simulink model "SD2231_Lab1_2022"  (R2020b)
settings: Solver=VariableStepAuto  StartTime=0.0  StopTime=inf  RelTol=1e-3
values from neighbouring files (symbols this model uses):
  delay = 250    [initial.m]
  K_awup = Ki_br_r/Kp_br_r    (= 10.4166666667)    [initial.m]
  K_brake = K_brake(3)    [initial.m]
  K_em = K_em(3)    [initial.m]
  Kd_br_f = 0*0.6*T_new_rl_b    (= 0)    [initial.m]
  Kd_br_r = 0.6*T_new_rl_b    (= 0.1722)    [initial.m]
  Kd_tr = 0.6*T_new    (= 0.0093)    [initial.m]
  Ki_br_f = 0.5*0.6*T_new_rl_b/L_new_rl_b^2    (= 37.3697916667)    [initial.m]
  Ki_br_r = 0.6*T_new_rl_b/L_new_rl_b^2    (= 74.7395833333)    [initial.m]
  Ki_tr = 0.6*T_new/L_new^2    (= 4.12188365651)    [initial.m]
  Kp_br_f = 1.2*T_new_rl_b/L_new_rl_b    (= 7.175)    [initial.m]
  Kp_br_r = 1.2*T_new_rl_b/L_new_rl_b    (= 7.175)    [initial.m]
  Kp_tr = 2.2*1.2*T_new/L_new    (= 0.861473684211)    [initial.m]
  N = 100    [initial.m]
  ref_br_f = 0.15    [initial.m]
  ref_br_r = 0.17-0.1    (= 0.07)    [initial.m]
  ref_tr = 0.06    [initial.m]
  step_time = 2    [initial.m]
  threshold_br_f = ref_br_f-0.05    (= 0.1)    [initial.m]
  threshold_br_r = ref_br_r-0.05    (= 0.02)    [initial.m]
  threshold_tc = ref_tr-0.02    (= 0.04)    [initial.m]
  vx_threshold = 1    [initial.m]
undefined symbols (not defined in the file or in its folder): DiscIntNeverNeededParam, Veh
libraries: CarMaker4SL x38, simulink x2, autolibmappedmotor x2
(part 1 of 4)
settings Model: Creator=Edwin solomon  LastModifiedBy=rivaa

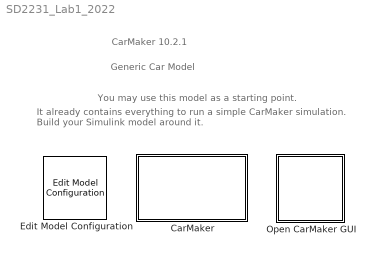
== system SD2231_Lab1_2022 ==
  note: You may use this model as a starting point.
  note: CarMaker 10.2.1
  note: It already contains everything to run a simple CarMaker simulation.
      | Build your Simulink model around it.
  note: Generic Car Model
  CarMaker : Subsystem  TreatAsAtomicUnit=on
      mask Display: image(imread('CarMakerSys.png'));
  Edit Model Configuration : CarMaker4SL/Edit Model Configuration  SFunctionModules=''
  Open CarMaker GUI : Subsystem  LoadFcn=if ~length(which('cmself')), cmenv; end
      settings: OpenFcn=cmblockmagic('gui_fix_display'); CM_Simulink
      mask Display: image(imread('CarMakerGUI.png'));

== system SD2231_Lab1_2022/CarMaker ==
  Bus Creator : BusCreator  Inputs=6
  CM_FIRST : Subsystem
  CM_LAST : Subsystem
  CarMaker data : Subsystem
  DrivMan : Subsystem
  Ground : Ground
  IPG Vehicle : Subsystem  TreatAsAtomicUnit=on
  Road friction : Subsystem
      settings: PortSchema="{\"entries\":[{\"content\":{\"sides\":[{\"content\":{\"connectorIds\":[]},\"type\":\"ConnectorPlacement.EquallySpacedRectSide\",\"uuid\":\"1e02911d-bb16-4af8-b063-0b1c76ab284f\"},{\"content\":{\"connectorIds\":[],\"side\":\"RIGHT\"},\"type\":\"ConnectorPlacement.EquallySpacedRectSide\",\"uuid\":\"1455e6df-1fb8-405b-9b14-078dc452472c\"},{\"content\":{\"connectorIds\":[\"In1\"],\"side\":\"TOP\"},\"type\":\"ConnectorPlacement.EquallySpacedRectSide\",\"uuid\":\"c8dda622-f685-4f5f-94e7-d49e41573b19\"},{\"content\":{\"connectorIds\":[],\"side\":\"HIDDEN\"},\"type\":\"ConnectorPlacement.EquallySpacedRectSide\",\"uuid\":\"9a4d84ea-b740-4dd8-ac4f-aa27e6a4f3a4\"}]},\"type\":\"ConnectorPlacement.EquallySpacedConnector\",\"uuid\":\"f3a55054-1857-4c4c-b5da-0ded36d4ade6\"}],\"packageUris\":[\"http://schema.mathworks.com/mf0/Connector/R2020b\"],\"version\":\"1.0\"}"
  Terminator : Terminator
  Used friction mapping : Subsystem
  VehicleControl : Subsystem
  Your ABS Controller : Subsystem
  Your Traction Controller : Subsystem
  Your observer : Subsystem
  wires:
  DrivMan/2(DrivMan.Out) -> VehicleControl/2(DrivMan.In)
  DrivMan/1(Sync_Out) -> VehicleControl/1(Sync_In)
  CM_FIRST/2(Env.Misc) -> DrivMan/2(Env.Misc)
  CM_FIRST/1(Sync_Out) -> DrivMan/1(Sync_In)
  CM_LAST/1(Sync_Out) -> Terminator/1
  Ground/1 -> CM_FIRST/1(Sync_In)
  IPG Vehicle/1(Sync_Out) -> CM_LAST/1(Sync_In)
  VehicleControl/1(Sync_Out) -> IPG Vehicle/1(Sync_In)
  VehicleControl/3(VhclCtrl.Steering) -> IPG Vehicle/3(VhclCtrl.Steering)
  VehicleControl/4(Vhcl.Wheel.In) -> IPG Vehicle/4(Vhcl.Wheel.In)
  VehicleControl/5(Vhcl.Misc) -> IPG Vehicle/5(Vhcl.Misc)
  VehicleControl/6(VhclCtrl.Brake) -> IPG Vehicle/6(VhclCtrl.Brake)
  VehicleControl/7(VhclCtrl.PT) -> IPG Vehicle/7(VhclCtrl.PT)
  VehicleControl/2(Vhcl.Model.Source) -> IPG Vehicle/2(Vhcl.Model.Source)
  Your Traction Controller/2(RR TrqReqSignal (0-1)) -> Bus Creator/2
  Your observer/2(Tyre slip bus data out) -> Your Traction Controller/2(Tyre slip bus data out), Used friction mapping/1(Tyre slip bus data out), Your ABS Controller/2(Tyre slip bus data out)
  Your observer/1(CarMaker bus data out) -> Your Traction Controller/1(CarMaker Bus data), Your ABS Controller/1(CarMaker Bus data)
  Your ABS Controller/3(RLBrakeAdjust (0-1)) -> Bus Creator/5
  CarMaker data/1(CarMaker bus data) -> Your observer/1(CarMaker bus data), Road friction/1(CarMaker bus data)
  Your ABS Controller/1(FLBrakeAdjust (0-1)) -> Bus Creator/3
  Your Traction Controller/1(LR TrqReqSignal (0-1)) -> Bus Creator/1
  Your ABS Controller/4(RRBrakeAdjust (0-1)) -> Bus Creator/6
  Bus Creator/1 -> IPG Vehicle/8(SD2231.data)
  Your ABS Controller/2(FRBrakeAdjust (0-1)) -> Bus Creator/4

== system SD2231_Lab1_2022/Open CarMaker GUI ==
  S-Function : S-Function  FunctionName=cm_gui  SFunctionDeploymentMode=off  EnableBusSupport=off

== system SD2231_Lab1_2022/CarMaker/CM_FIRST ==
  Sync_In : Inport
  BusCreator1 : BusCreator  Inputs=8
  BusCreator2 : BusCreator  Inputs=6
  Demux1 : Demux  Outputs=14
      settings: DisplayOption=none
  Environment : S-Function  FunctionName=CM_Sfun  Parameters='Environment'  SFunctionDeploymentMode=off  EnableBusSupport=off
  IoIn : S-Function  FunctionName=CM_Sfun  Parameters='IoIn'  SFunctionDeploymentMode=off  EnableBusSupport=off
  Terminator : Terminator
  Sync_Out : Outport
  Env.Misc : Outport  Port=2
  wires:
  BusCreator2/1 -> Terminator/1  "IF Environment (in)"
  BusCreator1/1 -> Env.Misc/1
  Demux1/14 -> BusCreator2/6  "Env sRoad"
  Demux1/13 -> BusCreator2/5  "Env PoI_GCS Elev"
  Demux1/12 -> BusCreator2/4  "Env PoI_GCS Lat"
  Demux1/11 -> BusCreator2/3  "Env PoI_GCS Long"
  Demux1/10 -> BusCreator2/2  "Env Time"
  Demux1/9 -> BusCreator2/1  "Env yDay"
  Demux1/8 -> BusCreator1/8  "Env WindVel_tot z"
  Demux1/7 -> BusCreator1/7  "Env WindVel_tot y"
  Demux1/6 -> BusCreator1/6  "Env WindVel_tot x"
  Demux1/5 -> BusCreator1/5  "Env SolarRadiation"
  Demux1/4 -> BusCreator1/4  "Env AirHumidity"
  Demux1/3 -> BusCreator1/3  "Env AirPressure"
  Demux1/2 -> BusCreator1/2  "Env AirDensity"
  Demux1/1 -> BusCreator1/1  "Env Temperature"
  Environment/2 -> Demux1/1
  Environment/1 -> Sync_Out/1
  IoIn/1 -> Environment/1
  Sync_In/1 -> IoIn/1

== system SD2231_Lab1_2022/CarMaker/CM_LAST ==
  Sync_In : Inport
  CM_User : S-Function  FunctionName=CM_Sfun  Parameters='CM_User'  SFunctionDeploymentMode=off  EnableBusSupport=off
  IoOut : S-Function  FunctionName=CM_Sfun  Parameters='IoOut'  SFunctionDeploymentMode=off  EnableBusSupport=off
  Sync_Out : Outport
  wires:
  IoOut/1 -> Sync_Out/1
  CM_User/1 -> IoOut/1
  Sync_In/1 -> CM_User/1

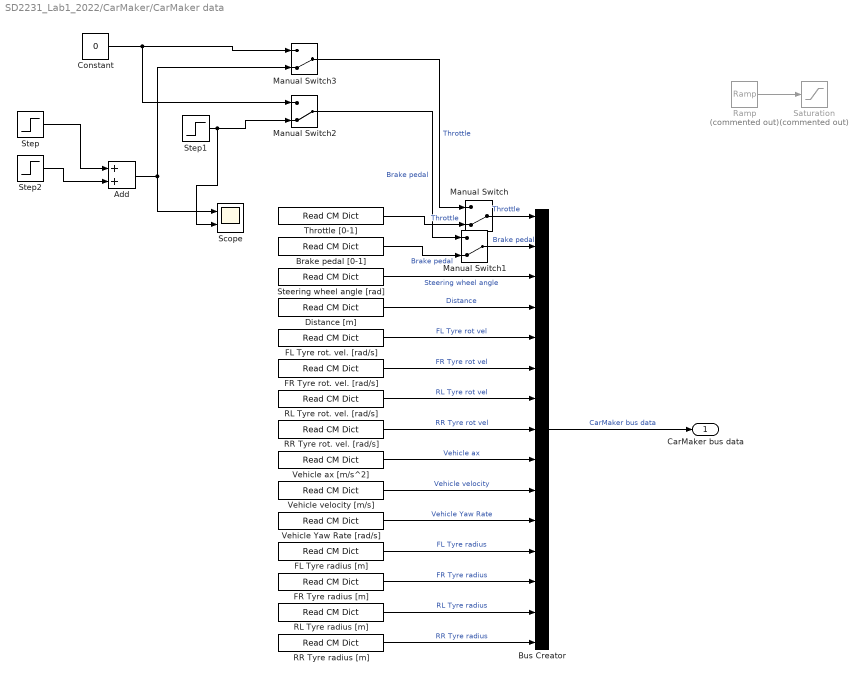
== system SD2231_Lab1_2022/CarMaker/CarMaker data ==
  Add : Sum
  Brake pedal [0-1] : CarMaker4SL/Read CM Dict  xname=Driver.Brake  xsync=off  xstime=Continuous
  Bus Creator : BusCreator  Inputs=15
  Constant : Constant  Value=0
  Distance [m] : CarMaker4SL/Read CM Dict  xname=Vhcl.Distance  xsync=off  xstime=Continuous
  FL Tyre radius [m] : CarMaker4SL/Read CM Dict  xname=Car.WFL.Radius  xsync=off  xstime=Continuous
  FL Tyre rot. vel. [rad/s] : CarMaker4SL/Read CM Dict  xname=Car.WheelSpd_FL  xsync=off  xstime=Continuous
  FR Tyre radius [m] : CarMaker4SL/Read CM Dict  xname=Car.WFR.Radius  xsync=off  xstime=Continuous
  FR Tyre rot. vel. [rad/s] : CarMaker4SL/Read CM Dict  xname=Car.WheelSpd_FR  xsync=off  xstime=Continuous
  Manual Switch{,1..3} (4 alike) : ManualSwitch  CurrentSetting=0
  RL Tyre radius [m] : CarMaker4SL/Read CM Dict  xname=Car.WRL.Radius  xsync=off  xstime=Continuous
  RL Tyre rot. vel. [rad/s] : CarMaker4SL/Read CM Dict  xname=Car.WheelSpd_RL  xsync=off  xstime=Continuous
  RR Tyre radius [m] : CarMaker4SL/Read CM Dict  xname=Car.WRR.Radius  xsync=off  xstime=Continuous
  RR Tyre rot. vel. [rad/s] : CarMaker4SL/Read CM Dict  xname=Car.WheelSpd_RR  xsync=off  xstime=Continuous
  Ramp : simulink/Sources/Ramp  Commented=on  slope=1/0.1  start=step_time  InitialOutput=0
  Saturation : Saturate  Commented=on  UpperLimit=1  LowerLimit=0
  Scope : Scope  NumInputPorts=2
  Steering wheel angle [rad] : CarMaker4SL/Read CM Dict  xname=Driver.Steer.Ang  xsync=off  xstime=Continuous
  Step : Step  Time=step_time  SampleTime=0
  Step1 : Step  Time=step_time + 6  SampleTime=0
  Step2 : Step  Time=step_time + 3  After=-1  SampleTime=0
  Throttle [0-1] : CarMaker4SL/Read CM Dict  xname=Driver.Gas  xsync=off  xstime=Continuous
  Vehicle Yaw Rate [rad/s] : CarMaker4SL/Read CM Dict  xname=Car.YawRate  xsync=off  xstime=Continuous
  Vehicle ax [m/s^2] : CarMaker4SL/Read CM Dict  xname=Car.ax  xsync=off  xstime=Continuous
  Vehicle velocity [m/s] : CarMaker4SL/Read CM Dict  xname=Car.v  xsync=off  xstime=Continuous
  CarMaker bus data : Outport  VectorParamsAs1DForOutWhenUnconnected=off
  wires:
  RR Tyre rot. vel. [rad/s]/1 -> Bus Creator/8  "RR Tyre rot vel"
  RL Tyre rot. vel. [rad/s]/1 -> Bus Creator/7  "RL Tyre rot vel"
  Distance [m]/1 -> Bus Creator/4  "Distance"
  FR Tyre rot. vel. [rad/s]/1 -> Bus Creator/6  "FR Tyre rot vel"
  Constant/1 -> Manual Switch2/1, Manual Switch3/1
  Vehicle ax [m/s^2]/1 -> Bus Creator/9  "Vehicle ax"
  Steering wheel angle [rad]/1 -> Bus Creator/3  "Steering wheel angle"
  Step/1 -> Add/1
  Vehicle velocity [m/s]/1 -> Bus Creator/10  "Vehicle velocity"
  FL Tyre rot. vel. [rad/s]/1 -> Bus Creator/5  "FL Tyre rot vel"
  Vehicle Yaw Rate [rad/s]/1 -> Bus Creator/11  "Vehicle Yaw Rate"
  FL Tyre radius [m]/1 -> Bus Creator/12  "FL Tyre radius"
  FR Tyre radius [m]/1 -> Bus Creator/13  "FR Tyre radius"
  RL Tyre radius [m]/1 -> Bus Creator/14  "RL Tyre radius"
  RR Tyre radius [m]/1 -> Bus Creator/15  "RR Tyre radius"
  Bus Creator/1 -> CarMaker bus data/1  "CarMaker bus data"
  Ramp/1 -> Saturation/1
  Manual Switch/1 -> Bus Creator/1  "Throttle"
  Manual Switch1/1 -> Bus Creator/2  "Brake pedal"
  Throttle [0-1]/1 -> Manual Switch/2  "Throttle"
  Brake pedal [0-1]/1 -> Manual Switch1/2  "Brake pedal"
  Manual Switch3/1 -> Manual Switch/1  "Throttle"
  Manual Switch2/1 -> Manual Switch1/1  "Brake pedal"
  Step1/1 -> Scope/2, Manual Switch2/2
  Step2/1 -> Add/2
  Add/1 -> Manual Switch3/2, Scope/1

== system SD2231_Lab1_2022/CarMaker/DrivMan ==
  note: There's rarely a reason to override DrivMan signals.
      | Use the VehicleControl interface for this purpose.
  Sync_In : Inport
  Env.Misc : Inport  Port=2
  BusCreator : BusCreator  Inputs=17
  Demux : Demux  Outputs=17
      settings: DisplayOption=none
  DrivMan : S-Function  FunctionName=CM_Sfun  Parameters='DrivMan'  SFunctionDeploymentMode=off  EnableBusSupport=off
  Sync_Out : Outport
  DrivMan.Out : Outport  Port=2
  wires:
  Demux/17 -> BusCreator/17  "DrivMan Steering Trq"
  Demux/16 -> BusCreator/16  "DrivMan Steering AngAcc"
  Demux/15 -> BusCreator/15  "DrivMan Steering AngVel"
  Demux/14 -> BusCreator/14  "DrivMan Steering Ang"
  Demux/13 -> BusCreator/13  "DrivMan Gas"
  Demux/12 -> BusCreator/12  "DrivMan Clutch"
  Demux/11 -> BusCreator/11  "DrivMan BrakePark"
  Demux/10 -> BusCreator/10  "DrivMan Brake"
  Demux/9 -> BusCreator/9  "DrivMan GearNo"
  Demux/8 -> BusCreator/8  "DrivMan SelectorCtrl"
  Demux/7 -> BusCreator/7  "DrivMan UserSignal4"
  Demux/6 -> BusCreator/6  "DrivMan UserSignal3"
  Demux/5 -> BusCreator/5  "DrivMan UserSignal2"
  Demux/4 -> BusCreator/4  "DrivMan UserSignal1"
  Demux/3 -> BusCreator/3  "DrivMan UserSignal0"
  Demux/2 -> BusCreator/2  "DrivMan Key"
  Demux/1 -> BusCreator/1  "DrivMan SST"
  Env.Misc/1 -> DrivMan/2
  Sync_In/1 -> DrivMan/1
  DrivMan/1 -> Sync_Out/1
  BusCreator/1 -> DrivMan.Out/1
  DrivMan/2 -> Demux/1

== system SD2231_Lab1_2022/CarMaker/IPG Vehicle ==
  Sync_In : Inport
  Vhcl.Model.Source : Inport  Port=2
  VhclCtrl.Steering : Inport  Port=3
  Vhcl.Wheel.In : Inport  Port=4
  Vhcl.Misc : Inport  Port=5
  VhclCtrl.Brake : Inport  Port=6
  VhclCtrl.PT : Inport  Port=7
  SD2231.data : Inport  Port=8
  Brake : Subsystem
  CarAndTrailer : Subsystem
  PowerTrain : Subsystem
  Stop Simulation : Stop
  VehicleSource_BuiltIn : simulink/Logic and Bit Operations/Compare To Constant  relop=~=  const=1  OutDataTypeStr=boolean  ZeroCross=off
  Sync_Out : Outport
  wires:
  VhclCtrl.PT/1 -> PowerTrain/3(VhclCtrl.PT)
  Brake/1(Sync_Out) -> PowerTrain/1(Sync_In)
  CarAndTrailer/1(Sync_Out) -> Brake/1(Sync_In)
  CarAndTrailer/2(Brake.IF.In) -> Brake/2(Brake.IF.In)
  VhclCtrl.Brake/1 -> Brake/3(VhclCtrl.Brake)
  PowerTrain/1(Sync_Out) -> Sync_Out/1
  Vhcl.Misc/1 -> CarAndTrailer/4(Vhcl.Misc)
  Vhcl.Wheel.In/1 -> CarAndTrailer/3(Vhcl.Wheel.In)
  VhclCtrl.Steering/1 -> CarAndTrailer/2(VhclCtrl.Steering)
  Sync_In/1 -> CarAndTrailer/1(Sync_In)
  Vhcl.Model.Source/1 -> VehicleSource_BuiltIn/1
  VehicleSource_BuiltIn/1 -> Stop Simulation/1
  Brake/2(Vhcl.Wheel.PT) -> PowerTrain/2(Vhcl.Wheel.PT)
  SD2231.data/1 -> PowerTrain/6(SD2232.data), Brake/4(SD2231.Data)
  Brake/3(Brake.IF.Out) -> PowerTrain/4(Brake.IF.Out)
  CarAndTrailer/3(Car.Trq_T2W) -> PowerTrain/5(Car.TrqT2W)

== system SD2231_Lab1_2022/CarMaker/Road friction ==
  CarMaker bus data : Inport
  Bus Selector : BusSelector  OutputSignals=Vehicle velocity,Vehicle ax
  Constant : Constant  Value=Veh.mu
  MATLAB Function : MATLAB Function  TreatAsAtomicUnit=on
  Manual Switch : ManualSwitch
  Scope : Scope  NumInputPorts=3
  Write CM Dict : CarMaker4SL/Write CM Dict  xname=Car.muRoadFL  xsync=off
  Write CM Dict1 : CarMaker4SL/Write CM Dict  xname=Car.muRoadFR  xsync=off
  Write CM Dict2 : CarMaker4SL/Write CM Dict  xname=Car.muRoadRL  xsync=off
  Write CM Dict3 : CarMaker4SL/Write CM Dict  xname=Car.muRoadRR  xsync=off
  wires:
  Manual Switch/1 -> Write CM Dict3/1, Write CM Dict2/1, Write CM Dict1/1, Write CM Dict/1
  MATLAB Function/1(mu) -> Manual Switch/1
  Constant/1 -> Manual Switch/2
  CarMaker bus data/1 -> Bus Selector/1
  Bus Selector/1 -> Scope/2, MATLAB Function/1(vx)  "<Vehicle velocity>"
  Bus Selector/2 -> Scope/3, MATLAB Function/2(ax)  "<Vehicle ax>"

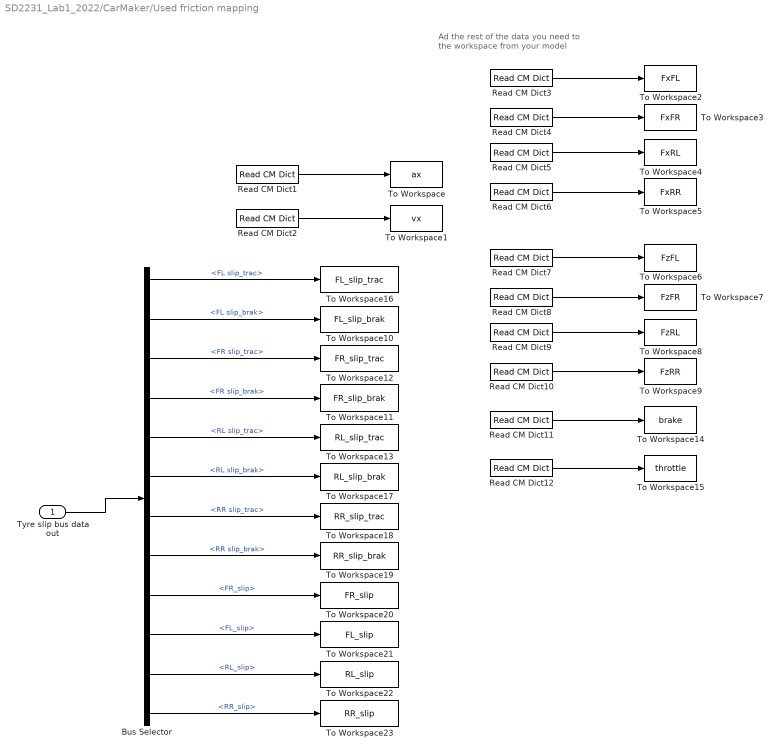
== system SD2231_Lab1_2022/CarMaker/Used friction mapping ==
  note: Ad the rest of the data you need to
      | the workspace from your model
  Tyre slip bus data out : Inport
  Bus Selector : BusSelector  OutputSignals=FL slip_trac,FL slip_brak,FR slip_trac,FR slip_brak,RL slip_trac,RL slip_brak,RR slip_trac,RR slip_brak,FR_slip,FL_slip,RL_slip,RR_slip
  Read CM Dict1 : CarMaker4SL/Read CM Dict  xname=Car.ax  xsync=off  xstime=Continuous
  Read CM Dict10 : CarMaker4SL/Read CM Dict  xname=Car.FzRR  xsync=off  xstime=Continuous
  Read CM Dict11 : CarMaker4SL/Read CM Dict  xname=Driver.Brake  xsync=off  xstime=Continuous
  Read CM Dict12 : CarMaker4SL/Read CM Dict  xname=Driver.Gas  xsync=off  xstime=Continuous
  Read CM Dict2 : CarMaker4SL/Read CM Dict  xname=Car.vx  xsync=off  xstime=Continuous
  Read CM Dict3 : CarMaker4SL/Read CM Dict  xname=Car.FxFL  xsync=off  xstime=Continuous
  Read CM Dict4 : CarMaker4SL/Read CM Dict  xname=Car.FxFR  xsync=off  xstime=Continuous
  Read CM Dict5 : CarMaker4SL/Read CM Dict  xname=Car.FxRL  xsync=off  xstime=Continuous
  Read CM Dict6 : CarMaker4SL/Read CM Dict  xname=Car.FxRR  xsync=off  xstime=Continuous
  Read CM Dict7 : CarMaker4SL/Read CM Dict  xname=Car.FzFL  xsync=off  xstime=Continuous
  Read CM Dict8 : CarMaker4SL/Read CM Dict  xname=Car.FzFR  xsync=off  xstime=Continuous
  Read CM Dict9 : CarMaker4SL/Read CM Dict  xname=Car.FzRL  xsync=off  xstime=Continuous
  To Workspace : ToWorkspace  VariableName=ax  SampleTime=-1
  To Workspace1 : ToWorkspace  VariableName=vx  SampleTime=-1
  To Workspace10 : ToWorkspace  VariableName=FL_slip_brak  SampleTime=-1
  To Workspace11 : ToWorkspace  VariableName=FR_slip_brak  SampleTime=-1
  To Workspace12 : ToWorkspace  VariableName=FR_slip_trac  SampleTime=-1
  To Workspace13 : ToWorkspace  VariableName=RL_slip_trac  SampleTime=-1
  To Workspace14 : ToWorkspace  VariableName=brake  SampleTime=-1
  To Workspace15 : ToWorkspace  VariableName=throttle  SampleTime=-1
  To Workspace16 : ToWorkspace  VariableName=FL_slip_trac  SampleTime=-1
  To Workspace17 : ToWorkspace  VariableName=RL_slip_brak  SampleTime=-1
  To Workspace18 : ToWorkspace  VariableName=RR_slip_trac  SampleTime=-1
  To Workspace19 : ToWorkspace  VariableName=RR_slip_brak  SampleTime=-1
  To Workspace2 : ToWorkspace  VariableName=FxFL  SampleTime=-1
  To Workspace20 : ToWorkspace  VariableName=FR_slip  SampleTime=-1
  To Workspace21 : ToWorkspace  VariableName=FL_slip  SampleTime=-1
  To Workspace22 : ToWorkspace  VariableName=RL_slip  SampleTime=-1
  To Workspace23 : ToWorkspace  VariableName=RR_slip  SampleTime=-1
  To Workspace3 : ToWorkspace  VariableName=FxFR  SampleTime=-1
  To Workspace4 : ToWorkspace  VariableName=FxRL  SampleTime=-1
  To Workspace5 : ToWorkspace  VariableName=FxRR  SampleTime=-1
  To Workspace6 : ToWorkspace  VariableName=FzFL  SampleTime=-1
  To Workspace7 : ToWorkspace  VariableName=FzFR  SampleTime=-1
  To Workspace8 : ToWorkspace  VariableName=FzRL  SampleTime=-1
  To Workspace9 : ToWorkspace  VariableName=FzRR  SampleTime=-1
  wires:
  Read CM Dict1/1 -> To Workspace/1
  Tyre slip bus data out/1 -> Bus Selector/1
  Read CM Dict2/1 -> To Workspace1/1
  Read CM Dict3/1 -> To Workspace2/1
  Read CM Dict4/1 -> To Workspace3/1
  Read CM Dict6/1 -> To Workspace5/1
  Read CM Dict5/1 -> To Workspace4/1
  Read CM Dict9/1 -> To Workspace8/1
  Read CM Dict10/1 -> To Workspace9/1
  Read CM Dict8/1 -> To Workspace7/1
  Read CM Dict7/1 -> To Workspace6/1
  Bus Selector/2 -> To Workspace10/1  "<FL slip_brak>"
  Bus Selector/4 -> To Workspace11/1  "<FR slip_brak>"
  Bus Selector/3 -> To Workspace12/1  "<FR slip_trac>"
  Bus Selector/5 -> To Workspace13/1  "<RL slip_trac>"
  Read CM Dict11/1 -> To Workspace14/1
  Read CM Dict12/1 -> To Workspace15/1
  Bus Selector/1 -> To Workspace16/1  "<FL slip_trac>"
  Bus Selector/6 -> To Workspace17/1  "<RL slip_brak>"
  Bus Selector/7 -> To Workspace18/1  "<RR slip_trac>"
  Bus Selector/8 -> To Workspace19/1  "<RR slip_brak>"
  Bus Selector/9 -> To Workspace20/1  "<FR_slip>"
  Bus Selector/12 -> To Workspace23/1  "<RR_slip>"
  Bus Selector/11 -> To Workspace22/1  "<RL_slip>"
  Bus Selector/10 -> To Workspace21/1  "<FL_slip>"

== system SD2231_Lab1_2022/CarMaker/VehicleControl ==
  note: <Your model here>
  note: When implementing a vehicle control model,
      | be sure to add '-disablevehiclecontrol' to the command line arguments
      | in the CarMaker Model Configuration block.
      | Otherwise your model will possibly not see the original DrivMan signals
      | on its inputs, but those of a currently activated C-coded vehicle control model instead.
  Sync_In : Inport
  DrivMan.In : Inport  Port=2
  Bus Creator2 : BusCreator  Inputs=2
  CreateBus Vhcl.Misc : Subsystem
  CreateBus Vhcl.Wheel.In : Subsystem
  CreateBus VhclCtrl : Subsystem
  CreateBus VhclCtrl.PT : Subsystem
  CreateBus VhclCtrl.Steering : Subsystem
  Demux2 : Demux  Outputs=2
      settings: DisplayOption=none
  VehicleControl : S-Function  FunctionName=CM_Sfun  Parameters='VehicleControl'  SFunctionDeploymentMode=off  EnableBusSupport=off
  VehicleControlUpd : S-Function  FunctionName=CM_Sfun  Parameters='VehicleControlUpd'  SFunctionDeploymentMode=off  EnableBusSupport=off
  Sync_Out : Outport
  Vhcl.Model.Source : Outport  Port=2
  VhclCtrl.Steering : Outport  Port=3
  Vhcl.Wheel.In : Outport  Port=4
  Vhcl.Misc : Outport  Port=5
  VhclCtrl.Brake : Outport  Port=6
  VhclCtrl.PT : Outport  Port=7
  wires:
  CreateBus VhclCtrl/1(Out) -> VehicleControlUpd/2
  VehicleControl/2 -> CreateBus VhclCtrl/1(In)
  VehicleControlUpd/2 -> Vhcl.Model.Source/1
  VehicleControlUpd/4 -> CreateBus Vhcl.Wheel.In/1(In1)
  VehicleControlUpd/5 -> CreateBus Vhcl.Misc/1(In1)
  VehicleControlUpd/6 -> Demux2/1
  VehicleControlUpd/7 -> CreateBus VhclCtrl.PT/1(In1)
  VehicleControlUpd/3 -> CreateBus VhclCtrl.Steering/1(In1)
  CreateBus Vhcl.Misc/1(Out1) -> Vhcl.Misc/1
  CreateBus Vhcl.Wheel.In/1(Out1) -> Vhcl.Wheel.In/1
  DrivMan.In/1 -> VehicleControl/2
  VehicleControl/1 -> VehicleControlUpd/1
  Sync_In/1 -> VehicleControl/1
  CreateBus VhclCtrl.PT/1(Out1) -> VhclCtrl.PT/1
  Bus Creator2/1 -> VhclCtrl.Brake/1
  CreateBus VhclCtrl.Steering/1(Out1) -> VhclCtrl.Steering/1
  VehicleControlUpd/1 -> Sync_Out/1
  Demux2/2 -> Bus Creator2/2  "VhclCtrl BrakePark"
  Demux2/1 -> Bus Creator2/1  "VhclCtrl Brake"

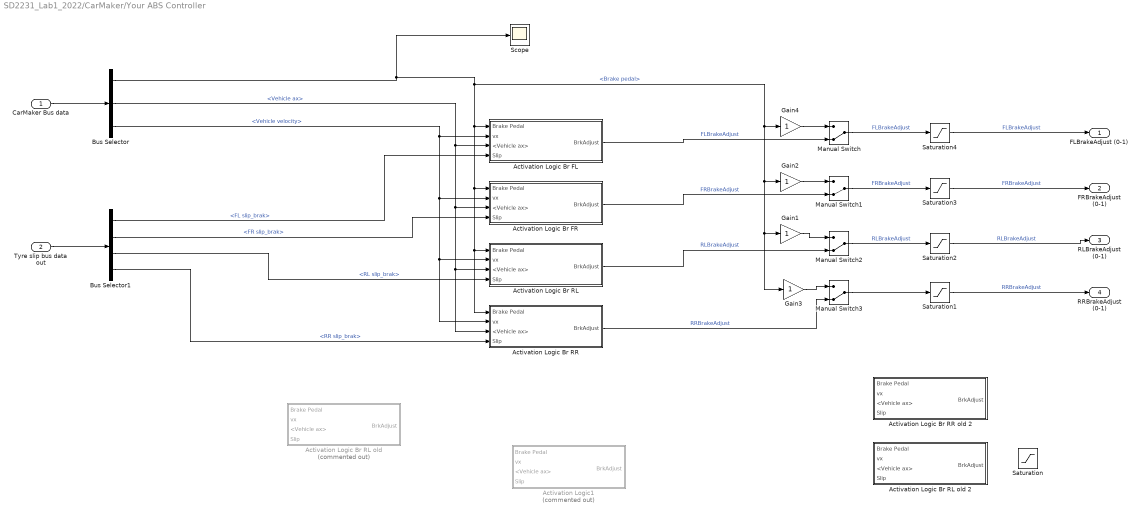
== system SD2231_Lab1_2022/CarMaker/Your ABS Controller ==
  CarMaker Bus data : Inport
  Tyre slip bus data out : Inport  Port=2
  Activation Logic Br FL : Subsystem
  Activation Logic Br FR : Subsystem
  Activation Logic Br RL : Subsystem
  Activation Logic Br RL old : Subsystem  Commented=on
  Activation Logic Br RL old 2 : Subsystem
  Activation Logic Br RR : Subsystem
  Activation Logic Br RR old 2 : Subsystem
  Activation Logic1 : Subsystem  Commented=on
  Bus Selector : BusSelector  OutputSignals=Brake pedal,Vehicle ax,Vehicle velocity
  Bus Selector1 : BusSelector  OutputSignals=FL slip_brak,FR slip_brak,RL slip_brak,RR slip_brak
  Gain{1..4} (4 alike) : Gain
  Manual Switch{,1..3} (4 alike) : ManualSwitch  CurrentSetting=0
  Saturation{,1..4} (5 alike) : Saturate  UpperLimit=1  LowerLimit=0
  Scope : Scope
  FLBrakeAdjust (0-1) : Outport  VectorParamsAs1DForOutWhenUnconnected=off
  FRBrakeAdjust (0-1) : Outport  Port=2  VectorParamsAs1DForOutWhenUnconnected=off
  RLBrakeAdjust (0-1) : Outport  Port=3  VectorParamsAs1DForOutWhenUnconnected=off
  RRBrakeAdjust (0-1) : Outport  Port=4  VectorParamsAs1DForOutWhenUnconnected=off
  wires:
  Bus Selector/1 -> Scope/1, Gain4/1, Gain2/1, Gain1/1, Gain3/1, Activation Logic Br FL/1(Brake Pedal), Activation Logic Br FR/1(Brake Pedal), Activation Logic Br RR/1(Brake Pedal), Activation Logic Br RL/1(Brake Pedal)  "<Brake pedal>"
  CarMaker Bus data/1 -> Bus Selector/1
  Tyre slip bus data out/1 -> Bus Selector1/1
  Bus Selector1/1 -> Activation Logic Br FL/4(" Slip")  "<FL slip_brak>"
  Bus Selector1/2 -> Activation Logic Br FR/4(" Slip")  "<FR slip_brak>"
  Bus Selector1/3 -> Activation Logic Br RL/4(" Slip")  "<RL slip_brak>"
  Bus Selector1/4 -> Activation Logic Br RR/4(" Slip")  "<RR slip_brak>"
  Activation Logic Br RL/1(BrkAdjust) -> Manual Switch2/2  "RLBrakeAdjust"
  Activation Logic Br FR/1(BrkAdjust) -> Manual Switch1/2  "FRBrakeAdjust"
  Activation Logic Br FL/1(BrkAdjust) -> Manual Switch/2  "FLBrakeAdjust"
  Manual Switch/1 -> Saturation4/1  "FLBrakeAdjust"
  Manual Switch1/1 -> Saturation3/1  "FRBrakeAdjust"
  Manual Switch2/1 -> Saturation2/1  "RLBrakeAdjust"
  Manual Switch3/1 -> Saturation1/1
  Gain2/1 -> Manual Switch1/1
  Gain3/1 -> Manual Switch3/1
  Gain1/1 -> Manual Switch2/1
  Gain4/1 -> Manual Switch/1
  Bus Selector/2 -> Activation Logic Br FL/3(<Vehicle ax>), Activation Logic Br FR/3(<Vehicle ax>), Activation Logic Br RR/3(<Vehicle ax>), Activation Logic Br RL/3(<Vehicle ax>)  "<Vehicle ax>"
  Bus Selector/3 -> Activation Logic Br FL/2(vx), Activation Logic Br FR/2(vx), Activation Logic Br RR/2(vx), Activation Logic Br RL/2(vx)  "<Vehicle velocity>"
  Activation Logic Br RR/1(BrkAdjust) -> Manual Switch3/2  "RRBrakeAdjust"
  Saturation1/1 -> RRBrakeAdjust (0-1)/1  "RRBrakeAdjust"
  Saturation2/1 -> RLBrakeAdjust (0-1)/1  "RLBrakeAdjust"
  Saturation3/1 -> FRBrakeAdjust (0-1)/1  "FRBrakeAdjust"
  Saturation4/1 -> FLBrakeAdjust (0-1)/1  "FLBrakeAdjust"

== system SD2231_Lab1_2022/CarMaker/Your Traction Controller ==
  CarMaker Bus data : Inport
  Tyre slip bus data out : Inport  Port=2
  Activation Logic RL tr1 : Subsystem  Commented=on
  Activation Logic RL tr2 : Subsystem  Commented=on
  Activation Logic Tr RL : Subsystem
  Activation Logic Tr RR : Subsystem
  Activation Logic1 : Subsystem
  Bus Selector : BusSelector  OutputSignals=Throttle,Vehicle ax
  Bus Selector1 : BusSelector  OutputSignals=RL slip_trac,RR slip_trac
  Gain : Gain
  Gain1 : Gain
  Manual Switch : ManualSwitch
  Manual Switch1 : ManualSwitch  CurrentSetting=0
  Saturation : Saturate  UpperLimit=1  LowerLimit=0
  Saturation1 : Saturate  UpperLimit=1  LowerLimit=0
  LR TrqReqSignal (0-1) : Outport  VectorParamsAs1DForOutWhenUnconnected=off
  RR TrqReqSignal (0-1) : Outport  Port=2  VectorParamsAs1DForOutWhenUnconnected=off
  wires:
  CarMaker Bus data/1 -> Bus Selector/1
  Tyre slip bus data out/1 -> Bus Selector1/1
  Bus Selector1/2 -> Activation Logic Tr RR/3(" Slip")  "<RR slip_trac>"
  Activation Logic Tr RL/1(RLTrqAdjust) -> Manual Switch/1  "LRTrqAdjust"
  Gain/1 -> Manual Switch/2
  Manual Switch/1 -> Saturation/1  "LRTrqAdjust"
  Activation Logic Tr RR/1(ThrAdjust) -> Manual Switch1/2
  Manual Switch1/1 -> Saturation1/1  "RRTrqAdjust"
  Saturation/1 -> LR TrqReqSignal (0-1)/1  "LRTrqAdjust"
  Saturation1/1 -> RR TrqReqSignal (0-1)/1  "RRTrqAdjust"
  Bus Selector/1 -> Activation Logic Tr RR/1(Thr), Gain1/1, Activation Logic Tr RL/1(<Throttle>), Gain/1  "<Throttle>"
  Bus Selector/2 -> Activation Logic Tr RR/2(<Vehicle ax>), Activation Logic Tr RL/2(ax)  "<Vehicle ax>"
  Bus Selector1/1 -> Activation Logic Tr RL/3(<RL Slip>)  "<RL slip_trac>"
  Gain1/1 -> Manual Switch1/1

== system SD2231_Lab1_2022/CarMaker/Your observer ==
  note: Ad your own slip observer
  CarMaker bus data : Inport
  Bus Selector : BusSelector  OutputSignals=Throttle,Brake pedal,Vehicle ax,Vehicle velocity
  Delay : Delay  DelayLength=200
  Scope : Scope  NumInputPorts=4
  Scope1 : Scope  NumInputPorts=2
  Slip observer : Subsystem
  CarMaker bus data out : Outport  VectorParamsAs1DForOutWhenUnconnected=off
  Tyre slip bus data out : Outport  Port=2  VectorParamsAs1DForOutWhenUnconnected=off
  wires:
  CarMaker bus data/1 -> Bus Selector/1, CarMaker bus data out/1, Slip observer/1(In1)
  Slip observer/1(Tyre slip bus out) -> Tyre slip bus data out/1
  Bus Selector/1 -> Delay/1, Scope1/2, Scope/1  "<Throttle>"
  Bus Selector/2 -> Scope/2  "<Brake pedal>"
  Bus Selector/3 -> Scope/3  "<Vehicle ax>"
  Bus Selector/4 -> Scope/4  "<Vehicle velocity>"
  Delay/1 -> Scope1/1

== system SD2231_Lab1_2022/CarMaker/IPG Vehicle/Brake ==
  note: When replacing the entire braking system,
      | be sure to disable the IPG brake model by using the brake
      | model 'Model Manager off' in the vehicle GUI.
  note: <Your model here>
  Sync_In : Inport
  Brake.IF.In : Inport  Port=2
  VhclCtrl.Brake : Inport  Port=3
  SD2231.Data : Inport  Port=4
  Brake : S-Function  FunctionName=CM_Sfun  Parameters='Brake'  SFunctionDeploymentMode=off  EnableBusSupport=off
  BrakeUpd : S-Function  FunctionName=CM_Sfun  Parameters='BrakeUpd'  SFunctionDeploymentMode=off  EnableBusSupport=off
  BusCreator1 : BusCreator  Inputs=16
  CreateBus Vhcl.Wheel.PT : Subsystem
  Demux : Demux  Outputs=16
      settings: DisplayOption=none
  Terminator : Terminator
  UserDefinedBrakingSystem : Subsystem  TreatAsAtomicUnit=on
  Sync_Out : Outport
  Vhcl.Wheel.PT : Outport  Port=2
  Brake.IF.Out : Outport  Port=3  VectorParamsAs1DForOutWhenUnconnected=off
  wires:
  Demux/16 -> BusCreator1/16  "Brake IF Trq_DriveSrc_trg d3"
  Demux/15 -> BusCreator1/15  "Brake IF Trq_DriveSrc_trg d2"
  Demux/14 -> BusCreator1/14  "Brake IF Trq_DriveSrc_trg d1"
  Demux/13 -> BusCreator1/13  "Brake IF Trq_DriveSrc_trg d0"
  Demux/12 -> BusCreator1/12  "Brake IF Trq_Reg_trg RR"
  Demux/11 -> BusCreator1/11  "Brake IF Trq_Reg_trg RL"
  Demux/10 -> BusCreator1/10  "Brake IF Trq_Reg_trg FR"
  Demux/9 -> BusCreator1/9  "Brake IF Trq_Reg_trg FL"
  Demux/8 -> BusCreator1/8  "Brake IF Trq_PB RR"
  Demux/7 -> BusCreator1/7  "Brake IF Trq_PB RL"
  Demux/6 -> BusCreator1/6  "Brake IF Trq_PB FR"
  Demux/5 -> BusCreator1/5  "Brake IF Trq_PB FL"
  Demux/4 -> BusCreator1/4  "Brake IF Trq_WB RR"
  Demux/3 -> BusCreator1/3  "Brake IF Trq_WB RL"
  Demux/2 -> BusCreator1/2  "Brake IF Trq_WB FR"
  Demux/1 -> BusCreator1/1  "Brake IF Trq_WB FL"
  Brake/2 -> Terminator/1
  BrakeUpd/1 -> Sync_Out/1
  Brake/1 -> BrakeUpd/1  "Sync"
  Brake.IF.In/1 -> Brake/2
  VhclCtrl.Brake/1 -> Brake/3
  Sync_In/1 -> Brake/1
  BrakeUpd/2 -> CreateBus Vhcl.Wheel.PT/1(In)
  CreateBus Vhcl.Wheel.PT/1(Out) -> Vhcl.Wheel.PT/1
  SD2231.Data/1 -> UserDefinedBrakingSystem/1(SD2231.Data)
  UserDefinedBrakingSystem/1(Brake.IF.Out) -> Demux/1
  BusCreator1/1 -> Brake.IF.Out/1, BrakeUpd/2

== system SD2231_Lab1_2022/CarMaker/IPG Vehicle/CarAndTrailer ==
  Sync_In : Inport
  VhclCtrl.Steering : Inport  Port=2
  Vhcl.Wheel.In : Inport  Port=3
  Vhcl.Misc : Inport  Port=4
  CarAndTrailerUpd : Subsystem
  Forces : Subsystem
  Ground : Ground
  Kinematics : Subsystem
  Kinetics : Subsystem
  Steering : Subsystem
  Terminator : Terminator
  Terminator1 : Terminator
  Trailer : Subsystem
  Sync_Out : Outport
  Brake.IF.In : Outport  Port=2
  Car.Trq_T2W : Outport  Port=3  VectorParamsAs1DForOutWhenUnconnected=off
  wires:
  Trailer/9(Car.Hitch.FrcTrq) -> CarAndTrailerUpd/9(Car.Hitch.FrcTrq)
  Trailer/8(Vhcl.Wheel.RR) -> CarAndTrailerUpd/8(Vhcl.Wheel.RR)
  Trailer/7(Vhcl.Wheel.RL) -> CarAndTrailerUpd/7(Vhcl.Wheel.RL)
  Trailer/6(Vhcl.Wheel.FR) -> CarAndTrailerUpd/6(Vhcl.Wheel.FR)
  Trailer/5(Vhcl.Wheel.FL) -> CarAndTrailerUpd/5(Vhcl.Wheel.FL)
  Trailer/4(Vhcl.PoI) -> CarAndTrailerUpd/4(Vhcl.PoI)
  Trailer/3(Vhcl.Motion) -> CarAndTrailerUpd/3(Vhcl.Motion)
  Trailer/2(Vhcl.Steering) -> CarAndTrailerUpd/2(Vhcl.Steering)
  Trailer/1(Sync_Out) -> CarAndTrailerUpd/1(Sync_In)
  CarAndTrailerUpd/2(Brake.IF.In) -> Brake.IF.In/1
  CarAndTrailerUpd/1(Sync_Out) -> Sync_Out/1
  Vhcl.Misc/1 -> Terminator1/1
  Vhcl.Wheel.In/1 -> Terminator/1
  Kinetics/6(WheelCarrier.Misc) -> Trailer/6(WheelCarrier.Misc)
  Kinetics/5(Car.Trq_T2W) -> Car.Trq_T2W/1, Trailer/5(Car.Trq_T2W)
  Steering/2(Steer.IF) -> Kinematics/2(Steer.IF)
  Kinetics/4(Car.Fr1) -> Trailer/4(Car.Fr1)
  Kinetics/3(Car.Hitch) -> Trailer/3(Car.Hitch)
  Kinetics/2(Trailer.Load) -> Trailer/2(Trailer.Load)
  VhclCtrl.Steering/1 -> Steering/2(VhclCtrl.Steering)
  Sync_In/1 -> Steering/1(Sync_In)
  Steering/1(Sync_Out) -> Kinematics/1(Sync_In)
  Kinetics/1(Sync_Out) -> Trailer/1(Sync_In)
  Ground/1 -> CarAndTrailerUpd/10(Vhcl.Fr1A)
  Forces/11(FStabi_ext) -> Kinetics/11(FStabi_ext)
  Forces/10(FDamp_ext) -> Kinetics/10(FDamp_ext)
  Forces/9(FSpring_ext) -> Kinetics/9(FSpring_ext)
  Forces/8(TireRR_Out) -> Kinetics/8(TireRR.Out)
  Forces/7(TireRL_Out) -> Kinetics/7(TireRL.Out)
  Forces/6(TireFR_Out) -> Kinetics/6(TireFR.Out)
  Forces/5(TireFL_Out) -> Kinetics/5(TireFL.Out)
  Forces/4(Car.Load) -> Kinetics/4(Car.Load)
  Forces/2(Car.Virtual) -> Kinetics/2(Car.Virtual)
  Kinematics/6(lSpring) -> Forces/6(lSpring)
  Kinematics/7(vDamp) -> Forces/7(vDamp)
  Forces/3(Car.Aero) -> Kinetics/3(Car.Aero)
  Forces/1(Sync_Out) -> Kinetics/1(Sync_In)
  Kinematics/5(TireRR_In) -> Forces/5(TireRR_In)
  Kinematics/4(TireRL_In) -> Forces/4(TireRL_In)
  Kinematics/3(TireFR_In) -> Forces/3(TireFR_In)
  Kinematics/2(TireFL_In) -> Forces/2(TireFL_In)
  Kinematics/1(Sync_Out) -> Forces/1(Sync_In)
  Kinematics/8(lStabi) -> Forces/8(lStabi)
  Forces/12(FBuf_ext) -> Kinetics/12(FBuf_ext)
  Kinematics/9(lBuf) -> Forces/9(lBuf)

== system SD2231_Lab1_2022/CarMaker/IPG Vehicle/PowerTrain ==
  note: When replacing the entire powertrain,
      | be sure to disable the IPG powertrain model by using the powertrain
      | model 'Model Manager off' in the vehicle GUI.
  note: <Your model here>
  Sync_In : Inport
  Vhcl.Wheel.PT : Inport  Port=2
  VhclCtrl.PT : Inport  Port=3
  Brake.IF.Out : Inport  Port=4
  Car.TrqT2W : Inport  Port=5
  SD2232.data : Inport  Port=6
  BusCreator1 : BusCreator  Inputs=42
  Demux1 : Demux  Outputs=42
      settings: DisplayOption=none
  PowerTrain : S-Function  FunctionName=CM_Sfun  Parameters='PowerTrain'  SFunctionDeploymentMode=off  EnableBusSupport=off
  PowerTrainUpd : S-Function  FunctionName=CM_Sfun  Parameters='PowerTrainUpd'  SFunctionDeploymentMode=off  EnableBusSupport=off
  Terminator : Terminator
  User RearDriven PowerTrain1 : Subsystem
  Sync_Out : Outport
  wires:
  BusCreator1/1 -> Terminator/1
  Demux1/42 -> BusCreator1/42  "PT IF WRR Trq_BrakeReg_max"
  Demux1/41 -> BusCreator1/41  "PT IF WRR Trq_BrakeReg"
  Demux1/40 -> BusCreator1/40  "PT IF WRR Trq_Supp2WC"
  Demux1/39 -> BusCreator1/39  "PT IF WRR Trq_Drive"
  Demux1/38 -> BusCreator1/38  "PT IF WRR Trq_B2W"
  Demux1/37 -> BusCreator1/37  "PT IF WRR rotv"
  Demux1/36 -> BusCreator1/36  "PT IF WRR rot"
  Demux1/35 -> BusCreator1/35  "PT IF WRL Trq_BrakeReg_max"
  Demux1/34 -> BusCreator1/34  "PT IF WRL Trq_BrakeReg"
  Demux1/33 -> BusCreator1/33  "PT IF WRL Trq_Supp2WC"
  Demux1/32 -> BusCreator1/32  "PT IF WRL Trq_Drive"
  Demux1/31 -> BusCreator1/31  "PT IF WRL Trq_B2W"
  Demux1/30 -> BusCreator1/30  "PT IF WRL rotv"
  Demux1/29 -> BusCreator1/29  "PT IF WRL rot"
  Demux1/28 -> BusCreator1/28  "PT IF WFR Trq_BrakeReg_max"
  Demux1/27 -> BusCreator1/27  "PT IF WFR Trq_BrakeReg"
  Demux1/26 -> BusCreator1/26  "PT IF WFR Trq_Supp2WC"
  Demux1/25 -> BusCreator1/25  "PT IF WFR Trq_Drive"
  Demux1/24 -> BusCreator1/24  "PT IF WFR Trq_B2W"
  Demux1/23 -> BusCreator1/23  "PT IF WFR rotv"
  Demux1/22 -> BusCreator1/22  "PT IF WFR rot"
  Demux1/21 -> BusCreator1/21  "PT IF WFL Trq_BrakeReg_max"
  Demux1/20 -> BusCreator1/20  "PT IF WFL Trq_BrakeReg"
  Demux1/19 -> BusCreator1/19  "PT IF WFL Trq_Supp2WC"
  Demux1/18 -> BusCreator1/18  "PT IF WFL Trq_Drive"
  Demux1/17 -> BusCreator1/17  "PT IF WFL Trq_B2W"
  Demux1/16 -> BusCreator1/16  "PT IF WFL rotv"
  Demux1/15 -> BusCreator1/15  "PT IF WFL rot"
  Demux1/14 -> BusCreator1/14  "PT IF DL_iDiff_mean"
  Demux1/13 -> BusCreator1/13  "PT IF Trq_Supp2BdyEng y"
  Demux1/12 -> BusCreator1/12  "PT IF Trq_Supp2BdyEng x"
  Demux1/11 -> BusCreator1/11  "PT IF Trq_Supp2Bdy1B z"
  Demux1/10 -> BusCreator1/10  "PT IF Trq_Supp2Bdy1B y"
  Demux1/9 -> BusCreator1/9  "PT IF Trq_Supp2Bdy1B x"
  Demux1/8 -> BusCreator1/8  "PT IF Trq_Supp2Bdy1 z"
  Demux1/7 -> BusCreator1/7  "PT IF Trq_Supp2Bdy1 y"
  Demux1/6 -> BusCreator1/6  "PT IF Trq_Supp2Bdy1 x"
  Demux1/5 -> BusCreator1/5  "PT IF Engine_rotv"
  Demux1/4 -> BusCreator1/4  "PT IF GearNo"
  Demux1/3 -> BusCreator1/3  "PT IF OperationError"
  Demux1/2 -> BusCreator1/2  "PT IF OperationState"
  Demux1/1 -> BusCreator1/1  "PT IF Ignition"
  Sync_In/1 -> PowerTrain/1
  PowerTrain/2 -> Demux1/1
  PowerTrainUpd/1 -> Sync_Out/1
  PowerTrain/1 -> PowerTrainUpd/1  "Sync"
  VhclCtrl.PT/1 -> User RearDriven PowerTrain1/1(VhclCtrl), PowerTrain/3
  Vhcl.Wheel.PT/1 -> PowerTrain/2
  Brake.IF.Out/1 -> User RearDriven PowerTrain1/2(BrakingTorques)
  Car.TrqT2W/1 -> User RearDriven PowerTrain1/3(ResistanceTorques)
  SD2232.data/1 -> User RearDriven PowerTrain1/4(SD2231.data)
  User RearDriven PowerTrain1/1(PowerTrainOut) -> PowerTrainUpd/2

== system SD2231_Lab1_2022/CarMaker/VehicleControl/CreateBus Vhcl.Misc ==
  In1 : Inport
  BusCreator : BusCreator  Inputs=11
  Demux : Demux  Outputs=11
      settings: DisplayOption=none
  Out1 : Outport
  wires:
  Demux/11 -> BusCreator/11  "Vhcl Wind_vel_0 z"
  Demux/10 -> BusCreator/10  "Vhcl Wind_vel_0 y"
  Demux/9 -> BusCreator/9  "Vhcl Wind_vel_0 x"
  Demux/8 -> BusCreator/8  "Vhcl Trq_DL2BdyEng y"
  Demux/7 -> BusCreator/7  "Vhcl Trq_DL2BdyEng x"
  Demux/6 -> BusCreator/6  "Vhcl Trq_DL2Bdy1B z"
  Demux/5 -> BusCreator/5  "Vhcl Trq_DL2Bdy1B y"
  Demux/4 -> BusCreator/4  "Vhcl Trq_DL2Bdy1B x"
  Demux/3 -> BusCreator/3  "Vhcl Trq_DL2Bdy1 z"
  Demux/2 -> BusCreator/2  "Vhcl Trq_DL2Bdy1 y"
  Demux/1 -> BusCreator/1  "Vhcl Trq_DL2Bdy1 x"
  In1/1 -> Demux/1
  BusCreator/1 -> Out1/1

== system SD2231_Lab1_2022/CarMaker/VehicleControl/CreateBus Vhcl.Wheel.In ==
  In1 : Inport
  Bus Creator1 : BusCreator  Inputs=12
  Demux1 : Demux  Outputs=12
      settings: DisplayOption=none
  Out1 : Outport
  wires:
  Demux1/12 -> Bus Creator1/12  "Vhcl Wheel RR rotv"
  Demux1/11 -> Bus Creator1/11  "Vhcl Wheel RR Trq_DL2WC"
  Demux1/10 -> Bus Creator1/10  "Vhcl Wheel RR Trq_B2WC"
  Demux1/9 -> Bus Creator1/9  "Vhcl Wheel RL rotv"
  Demux1/8 -> Bus Creator1/8  "Vhcl Wheel RL Trq_DL2WC"
  Demux1/7 -> Bus Creator1/7  "Vhcl Wheel RL Trq_B2WC"
  Demux1/6 -> Bus Creator1/6  "Vhcl Wheel FR rotv"
  Demux1/5 -> Bus Creator1/5  "Vhcl Wheel FR Trq_DL2WC"
  Demux1/4 -> Bus Creator1/4  "Vhcl Wheel FR Trq_B2WC"
  Demux1/3 -> Bus Creator1/3  "Vhcl Wheel FL rotv"
  In1/1 -> Demux1/1
  Bus Creator1/1 -> Out1/1
  Demux1/2 -> Bus Creator1/2  "Vhcl Wheel FL Trq_DL2WC"
  Demux1/1 -> Bus Creator1/1  "Vhcl Wheel FL Trq_B2WC"

== system SD2231_Lab1_2022/CarMaker/VehicleControl/CreateBus VhclCtrl ==
  In : Inport
  BusCreator : BusCreator  Inputs=29
  Demux : Demux  Outputs=29
      settings: DisplayOption=none
  Out : Outport
  wires:
  In/1 -> Demux/1
  BusCreator/1 -> Out/1
  Demux/1 -> BusCreator/1  "VhclCtrl SST"
  Demux/2 -> BusCreator/2  "VhclCtrl Key"
  Demux/3 -> BusCreator/3  "VhclCtrl UserSignal0"
  Demux/4 -> BusCreator/4  "VhclCtrl UserSignal1"
  Demux/5 -> BusCreator/5  "VhclCtrl UserSignal2"
  Demux/6 -> BusCreator/6  "VhclCtrl UserSignal3"
  Demux/7 -> BusCreator/7  "VhclCtrl UserSignal4"
  Demux/8 -> BusCreator/8  "VhclCtrl GearNo"
  Demux/9 -> BusCreator/9  "VhclCtrl SelectorCtrl"
  Demux/10 -> BusCreator/10  "VhclCtrl Brake"
  Demux/11 -> BusCreator/11  "VhclCtrl BrakePark"
  Demux/12 -> BusCreator/12  "VhclCtrl Clutch"
  Demux/13 -> BusCreator/13  "VhclCtrl Gas"
  Demux/14 -> BusCreator/14  "VhclCtrl Steering Ang"
  Demux/15 -> BusCreator/15  "VhclCtrl Steering AngVel"
  Demux/16 -> BusCreator/16  "VhclCtrl Steering AngAcc"
  Demux/17 -> BusCreator/17  "VhclCtrl Steering Trq"
  Demux/18 -> BusCreator/18  "VhclCtrl Lights LowBeam"
  Demux/19 -> BusCreator/19  "VhclCtrl Lights HighBeam"
  Demux/20 -> BusCreator/20  "VhclCtrl Lights Daytime"
  Demux/21 -> BusCreator/21  "VhclCtrl Lights ParkL"
  Demux/22 -> BusCreator/22  "VhclCtrl Lights ParkR"
  Demux/23 -> BusCreator/23  "VhclCtrl Lights IndL"
  Demux/24 -> BusCreator/24  "VhclCtrl Lights IndR"
  Demux/25 -> BusCreator/25  "VhclCtrl Lights FogFrontL"
  Demux/26 -> BusCreator/26  "VhclCtrl Lights FogFrontR"
  Demux/27 -> BusCreator/27  "VhclCtrl Lights FogRear"
  Demux/28 -> BusCreator/28  "VhclCtrl Lights Brake"
  Demux/29 -> BusCreator/29  "VhclCtrl Lights Reverse"

== system SD2231_Lab1_2022/CarMaker/VehicleControl/CreateBus VhclCtrl.PT ==
  In1 : Inport
  BusCreator1 : BusCreator  Inputs=12
  Demux1 : Demux  Outputs=12
      settings: DisplayOption=none
  Out1 : Outport
  wires:
  Demux1/12 -> BusCreator1/12  "VhclCtrl Brake"
  Demux1/11 -> BusCreator1/11  "VhclCtrl Gas"
  Demux1/10 -> BusCreator1/10  "VhclCtrl Clutch"
  Demux1/9 -> BusCreator1/9  "VhclCtrl SelectorCtrl"
  Demux1/8 -> BusCreator1/8  "VhclCtrl GearNo"
  Demux1/7 -> BusCreator1/7  "VhclCtrl UserSignal4"
  Demux1/6 -> BusCreator1/6  "VhclCtrl UserSignal3"
  Demux1/5 -> BusCreator1/5  "VhclCtrl UserSignal2"
  Demux1/4 -> BusCreator1/4  "VhclCtrl UserSignal1"
  Demux1/3 -> BusCreator1/3  "VhclCtrl UserSignal0"
  Demux1/2 -> BusCreator1/2  "VhclCtrl Key"
  Demux1/1 -> BusCreator1/1  "VhclCtrl SST"
  In1/1 -> Demux1/1
  BusCreator1/1 -> Out1/1

== system SD2231_Lab1_2022/CarMaker/VehicleControl/CreateBus VhclCtrl.Steering ==
  In1 : Inport
  Bus Creator : BusCreator  Inputs=5
  Demux : Demux  Outputs=5
      settings: DisplayOption=none
  Out1 : Outport
  wires:
  In1/1 -> Demux/1
  Bus Creator/1 -> Out1/1
  Demux/1 -> Bus Creator/1  "VhclCtrl Steering Ang"
  Demux/5 -> Bus Creator/5  "VhclCtrl Steering SteerByTrq"
  Demux/3 -> Bus Creator/3  "VhclCtrl Steering AngAcc"
  Demux/2 -> Bus Creator/2  "VhclCtrl Steering AngVel"
  Demux/4 -> Bus Creator/4  "VhclCtrl Steering Trq"

== system SD2231_Lab1_2022/CarMaker/Your ABS Controller/Activation Logic Br FL ==
  Brake Pedal : Inport
  vx : Inport  Port=2
  <Vehicle ax> : Inport  Port=3
  " Slip" : Inport  Port=4
  AdjBr FL : Scope  NumInputPorts=2
  Constant : Constant  Value=threshold_br_f
  Constant1 : Constant  Value=vx_threshold
  MATLAB Function : MATLAB Function  TreatAsAtomicUnit=on
  Subsystem : Subsystem
      settings: PortSchema="{\"entries\":[{\"content\":{\"sides\":[{\"content\":{\"connectorIds\":[\"In1\",\"In2\"]},\"type\":\"ConnectorPlacement.EquallySpacedRectSide\",\"uuid\":\"5cbd211e-f9c8-43f4-83d7-871b04fe90ea\"},{\"content\":{\"connectorIds\":[\"Out1\"],\"side\":\"RIGHT\"},\"type\":\"ConnectorPlacement.EquallySpacedRectSide\",\"uuid\":\"7fa8af9f-7b9f-4089-80e3-a9aa0072d831\"},{\"content\":{\"connectorIds\":[\"In3\"],\"side\":\"TOP\"},\"type\":\"ConnectorPlacement.EquallySpacedRectSide\",\"uuid\":\"e4a0fb24-cce3-4d5d-8c82-dcee69222b7b\"},{\"content\":{\"connectorIds\":[],\"side\":\"HIDDEN\"},\"type\":\"ConnectorPlacement.EquallySpacedRectSide\",\"uuid\":\"1dbaf2b9-056b-4908-bf5e-3fea819f12fb\"}]},\"type\":\"ConnectorPlacement.EquallySpacedConnector\",\"uuid\":\"c1423465-905b-4b91-a244-d319c117cff2\"}],\"packageUris\":[\"http://schema.mathworks.com/mf0/Connector/R2020b\"],\"version\":\"1.0\"}"
  ref : Constant  Value=ref_br_f
  BrkAdjust : Outport
  wires:
  vx/1 -> MATLAB Function/1(vx)
  <Vehicle ax>/1 -> MATLAB Function/2(ax)
  Constant/1 -> MATLAB Function/6(threshold)
  Brake Pedal/1 -> AdjBr FL/2, Subsystem/3(Brake Pedal), MATLAB Function/3(Brk)
  " Slip"/1 -> Subsystem/1(slip), MATLAB Function/4(slip)
  Subsystem/1(AdjThr) -> MATLAB Function/5(AdjBrk)
  MATLAB Function/1(y) -> AdjBr FL/1, BrkAdjust/1
  ref/1 -> Subsystem/2(ref_slip)
  Constant1/1 -> MATLAB Function/7(vx_threshold)

== system SD2231_Lab1_2022/CarMaker/Your ABS Controller/Activation Logic Br FR ==
  Brake Pedal : Inport
  vx : Inport  Port=2
  <Vehicle ax> : Inport  Port=3
  " Slip" : Inport  Port=4
  AdjBr FR : Scope
  Constant : Constant  Value=threshold_br_f
  Constant1 : Constant  Value=vx_threshold
  MATLAB Function : MATLAB Function  TreatAsAtomicUnit=on
  Subsystem : Subsystem  Commented=on
      settings: PortSchema="{\"entries\":[{\"content\":{\"sides\":[{\"content\":{\"connectorIds\":[\"In1\",\"In2\"]},\"type\":\"ConnectorPlacement.EquallySpacedRectSide\",\"uuid\":\"5cec5cc2-4d6d-4b1d-b966-22042b341a0b\"},{\"content\":{\"connectorIds\":[\"Out1\"],\"side\":\"RIGHT\"},\"type\":\"ConnectorPlacement.EquallySpacedRectSide\",\"uuid\":\"00dd4905-e656-4dce-9ac4-4fe3f823c1f7\"},{\"content\":{\"connectorIds\":[\"In3\"],\"side\":\"TOP\"},\"type\":\"ConnectorPlacement.EquallySpacedRectSide\",\"uuid\":\"696fd126-3e4c-4262-b5bc-c3625537c515\"},{\"content\":{\"connectorIds\":[],\"side\":\"HIDDEN\"},\"type\":\"ConnectorPlacement.EquallySpacedRectSide\",\"uuid\":\"3dd45ed5-25e2-4347-abdf-21481b15662e\"}]},\"type\":\"ConnectorPlacement.EquallySpacedConnector\",\"uuid\":\"5000242c-67c6-4855-a207-79a064e97cc6\"}],\"packageUris\":[\"http://schema.mathworks.com/mf0/Connector/R2020b\"],\"version\":\"1.0\"}"
  Subsystem1 : Subsystem
      settings: PortSchema="{\"entries\":[{\"content\":{\"sides\":[{\"content\":{\"connectorIds\":[\"In1\",\"In2\"]},\"type\":\"ConnectorPlacement.EquallySpacedRectSide\",\"uuid\":\"5cec5cc2-4d6d-4b1d-b966-22042b341a0b\"},{\"content\":{\"connectorIds\":[\"Out1\"],\"side\":\"RIGHT\"},\"type\":\"ConnectorPlacement.EquallySpacedRectSide\",\"uuid\":\"00dd4905-e656-4dce-9ac4-4fe3f823c1f7\"},{\"content\":{\"connectorIds\":[\"In3\"],\"side\":\"TOP\"},\"type\":\"ConnectorPlacement.EquallySpacedRectSide\",\"uuid\":\"696fd126-3e4c-4262-b5bc-c3625537c515\"},{\"content\":{\"connectorIds\":[],\"side\":\"HIDDEN\"},\"type\":\"ConnectorPlacement.EquallySpacedRectSide\",\"uuid\":\"3dd45ed5-25e2-4347-abdf-21481b15662e\"}]},\"type\":\"ConnectorPlacement.EquallySpacedConnector\",\"uuid\":\"5000242c-67c6-4855-a207-79a064e97cc6\"}],\"packageUris\":[\"http://schema.mathworks.com/mf0/Connector/R2020b\"],\"version\":\"1.0\"}"
  ref : Constant  Value=ref_br_f
  BrkAdjust : Outport
  wires:
  ref/1 -> Subsystem1/2(ref_slip)
  MATLAB Function/1(y) -> AdjBr FR/1, BrkAdjust/1
  Subsystem1/1(AdjThr) -> MATLAB Function/5(AdjBrk)
  " Slip"/1 -> Subsystem1/1(slip), MATLAB Function/4(slip)
  Brake Pedal/1 -> Subsystem1/3(Brake Pedal), MATLAB Function/3(Brk)
  Constant/1 -> MATLAB Function/6(threshold)
  <Vehicle ax>/1 -> MATLAB Function/2(ax)
  vx/1 -> MATLAB Function/1(vx)
  Constant1/1 -> MATLAB Function/7(vx_threshold)

== system SD2231_Lab1_2022/CarMaker/Your ABS Controller/Activation Logic Br RL ==
  Brake Pedal : Inport
  vx : Inport  Port=2
  <Vehicle ax> : Inport  Port=3
  " Slip" : Inport  Port=4
  AdjBr RL : Scope  NumInputPorts=2
  Constant : Constant  Value=threshold_br_r
  Constant1 : Constant  Value=vx_threshold
  MATLAB Function : MATLAB Function  TreatAsAtomicUnit=on
  Subsystem : Subsystem
      settings: PortSchema="{\"entries\":[{\"content\":{\"sides\":[{\"content\":{\"connectorIds\":[\"In1\",\"In2\"]},\"type\":\"ConnectorPlacement.EquallySpacedRectSide\",\"uuid\":\"5cbd211e-f9c8-43f4-83d7-871b04fe90ea\"},{\"content\":{\"connectorIds\":[\"Out1\"],\"side\":\"RIGHT\"},\"type\":\"ConnectorPlacement.EquallySpacedRectSide\",\"uuid\":\"7fa8af9f-7b9f-4089-80e3-a9aa0072d831\"},{\"content\":{\"connectorIds\":[\"In3\"],\"side\":\"TOP\"},\"type\":\"ConnectorPlacement.EquallySpacedRectSide\",\"uuid\":\"e4a0fb24-cce3-4d5d-8c82-dcee69222b7b\"},{\"content\":{\"connectorIds\":[],\"side\":\"HIDDEN\"},\"type\":\"ConnectorPlacement.EquallySpacedRectSide\",\"uuid\":\"1dbaf2b9-056b-4908-bf5e-3fea819f12fb\"}]},\"type\":\"ConnectorPlacement.EquallySpacedConnector\",\"uuid\":\"c1423465-905b-4b91-a244-d319c117cff2\"}],\"packageUris\":[\"http://schema.mathworks.com/mf0/Connector/R2020b\"],\"version\":\"1.0\"}"
  ref : Constant  Value=ref_br_r
  BrkAdjust : Outport
  wires:
  vx/1 -> MATLAB Function/1(vx)
  <Vehicle ax>/1 -> MATLAB Function/2(ax)
  Constant/1 -> MATLAB Function/6(threshold)
  Brake Pedal/1 -> AdjBr RL/2, Subsystem/3(Brake Pedal), MATLAB Function/3(Brk)
  " Slip"/1 -> Subsystem/1(slip), MATLAB Function/4(slip)
  Subsystem/1(AdjThr) -> MATLAB Function/5(AdjBrk)
  MATLAB Function/1(y) -> AdjBr RL/1, BrkAdjust/1
  ref/1 -> Subsystem/2(ref_slip)
  Constant1/1 -> MATLAB Function/7(vx_threshold)

== system SD2231_Lab1_2022/CarMaker/Your ABS Controller/Activation Logic Br RL old ==
  Brake Pedal : Inport
  vx : Inport  Port=2
  <Vehicle ax> : Inport  Port=3
  " Slip" : Inport  Port=4
  AdjBrk RL : Scope
  Constant : Constant  Value=threshold_br_r
  Constant1 : Constant  Value=vx_threshold
  MATLAB Function : MATLAB Function  TreatAsAtomicUnit=on
  Subsystem : Subsystem
      settings: PortSchema="{\"entries\":[{\"content\":{\"sides\":[{\"content\":{\"connectorIds\":[\"In1\",\"In2\"]},\"type\":\"ConnectorPlacement.EquallySpacedRectSide\",\"uuid\":\"5cec5cc2-4d6d-4b1d-b966-22042b341a0b\"},{\"content\":{\"connectorIds\":[\"Out1\"],\"side\":\"RIGHT\"},\"type\":\"ConnectorPlacement.EquallySpacedRectSide\",\"uuid\":\"00dd4905-e656-4dce-9ac4-4fe3f823c1f7\"},{\"content\":{\"connectorIds\":[\"In3\"],\"side\":\"TOP\"},\"type\":\"ConnectorPlacement.EquallySpacedRectSide\",\"uuid\":\"696fd126-3e4c-4262-b5bc-c3625537c515\"},{\"content\":{\"connectorIds\":[],\"side\":\"HIDDEN\"},\"type\":\"ConnectorPlacement.EquallySpacedRectSide\",\"uuid\":\"3dd45ed5-25e2-4347-abdf-21481b15662e\"}]},\"type\":\"ConnectorPlacement.EquallySpacedConnector\",\"uuid\":\"5000242c-67c6-4855-a207-79a064e97cc6\"}],\"packageUris\":[\"http://schema.mathworks.com/mf0/Connector/R2020b\"],\"version\":\"1.0\"}"
  ref : Constant  Value=ref_br_r
  BrkAdjust : Outport
  wires:
  ref/1 -> Subsystem/2(ref_slip)
  MATLAB Function/1(y) -> AdjBrk RL/1, BrkAdjust/1
  Subsystem/1(AdjThr) -> MATLAB Function/5(AdjBrk)
  " Slip"/1 -> MATLAB Function/4(slip), Subsystem/1(slip)
  Brake Pedal/1 -> Subsystem/3(Brake Pedal), MATLAB Function/3(Brk)
  Constant/1 -> MATLAB Function/6(threshold)
  <Vehicle ax>/1 -> MATLAB Function/2(ax)
  vx/1 -> MATLAB Function/1(vx)
  Constant1/1 -> MATLAB Function/7(vx_threshold)

== system SD2231_Lab1_2022/CarMaker/Your ABS Controller/Activation Logic Br RL old 2 ==
  Brake Pedal : Inport
  vx : Inport  Port=2
  <Vehicle ax> : Inport  Port=3
  " Slip" : Inport  Port=4
  Constant : Constant  Value=threshold_br_r
  Constant1 : Constant  Value=vx_threshold
  Controller : Subsystem
      settings: PortSchema="{\"entries\":[{\"content\":{\"sides\":[{\"content\":{\"connectorIds\":[\"In1\",\"In2\"]},\"type\":\"ConnectorPlacement.EquallySpacedRectSide\",\"uuid\":\"5cec5cc2-4d6d-4b1d-b966-22042b341a0b\"},{\"content\":{\"connectorIds\":[\"Out1\"],\"side\":\"RIGHT\"},\"type\":\"ConnectorPlacement.EquallySpacedRectSide\",\"uuid\":\"00dd4905-e656-4dce-9ac4-4fe3f823c1f7\"},{\"content\":{\"connectorIds\":[\"In3\"],\"side\":\"TOP\"},\"type\":\"ConnectorPlacement.EquallySpacedRectSide\",\"uuid\":\"696fd126-3e4c-4262-b5bc-c3625537c515\"},{\"content\":{\"connectorIds\":[],\"side\":\"HIDDEN\"},\"type\":\"ConnectorPlacement.EquallySpacedRectSide\",\"uuid\":\"3dd45ed5-25e2-4347-abdf-21481b15662e\"}]},\"type\":\"ConnectorPlacement.EquallySpacedConnector\",\"uuid\":\"5000242c-67c6-4855-a207-79a064e97cc6\"}],\"packageUris\":[\"http://schema.mathworks.com/mf0/Connector/R2020b\"],\"version\":\"1.0\"}"
  MATLAB Function : MATLAB Function  TreatAsAtomicUnit=on
  Scope : Scope
  Switch : Switch  Commented=on  Criteria=u2 > Threshold  Threshold=5
  ref : Constant  Value=ref_br_r
  ref1 : Constant  Commented=on  Value=0
  BrkAdjust : Outport
  wires:
  ref1/1 -> Switch/3
  Switch/1 -> ?
  ? -> Switch/2
  Constant1/1 -> MATLAB Function/7(vx_threshold)
  vx/1 -> MATLAB Function/1(vx)
  ref/1 -> Controller/2(ref_slip)
  MATLAB Function/1(y) -> BrkAdjust/1, Scope/1
  Controller/1(AdjThr) -> MATLAB Function/5(AdjBrk)
  " Slip"/1 -> MATLAB Function/4(slip), Controller/1(slip)
  Brake Pedal/1 -> MATLAB Function/3(Brk), Controller/3(Brake Pedal)
  Constant/1 -> MATLAB Function/6(threshold)
  <Vehicle ax>/1 -> MATLAB Function/2(ax)
